simulink model "DWT_opt_fixed_point"  (R2022b)
settings: Solver=VariableStepAuto  StartTime=0.0  StopTime=st*279+st*length(signalx)  RelTol=1e-3
undefined symbols (not defined in the file): st, xc7z020clg484
libraries: hdlBasic x690, vmcUtilities x1
(part 1 of 3)
settings Model: Creator=SHMLab  LastModifiedBy=alanh

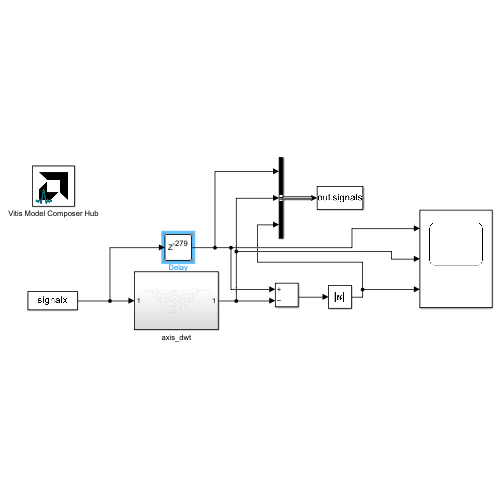
[thumbnail: Simulink's stored preview of the top-level diagram]
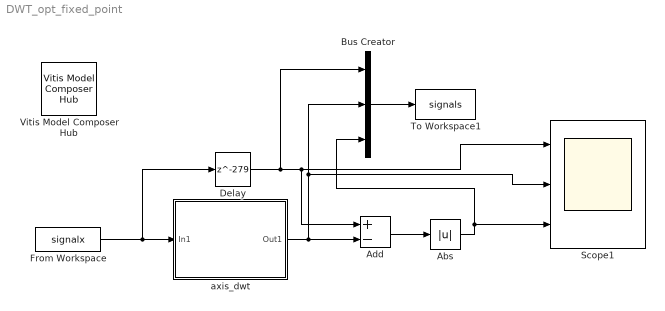
== system DWT_opt_fixed_point ==
  Abs : Abs  SaturateOnIntegerOverflow=off
  Add : Sum  Inputs=+-
  Bus Creator : BusCreator  Inputs=3
  Delay : Delay  DelayLength=279  InitialCondition=0
  From Workspace : FromWorkspace  VariableName=signalx  SampleTime=st  Interpolate=off  OutputAfterFinalValue=Setting to zero
  Scope1 : Scope  NumInputPorts=3
  To Workspace1 : ToWorkspace  VariableName=signals  SaveFormat=Timeseries  SampleTime=-1
      settings: Save2DSignal=2-D array (concatenate along first dimension)
  Vitis Model Composer Hub : vmcUtilities/Vitis Model Composer Hub  Tag=genX  CodeGeneration=off  SubsystemName=axis_dwt  TargetDirectory=./code  ExportType=HDL  IpVendor=xilinx.com  IpLibrary=hls  IpVersion=1.0  IpHWLanguage=Verilog  AieCompilerOptions={}  AieSimulatorOptions={}  CreateTestbench=off  TestbenchStackSize=10  RunRtlSim=off  RunCSim=off  RunAieSim=off  AieSimTimeout=50000  RunAieSimProfiling=off  LaunchVitisAnalyzer=off  PlotOutput=off  RunX86Sim=off  X86SimTimeout=10  GenHwImage=off  GenLibadfXo=off  PlatformType=Not Specified  HwSystemType=Baremetal  HwValidationTarget=hw  ProjDevice=xc7z020clg484-1  ProjDevicePart=xc7z020clg484-1  AIEType=None  SamplePeriod=-1  ClockFrequency=200  DataPathParallelism=1  xilinxfamily=zynq  part=xc7z020  speed=-1  package=clg484  directory=C:/Users/alanh/Downloads/Thesis/vivado/ip_with_clk_en\ip\axis_dwt\src  testbench=off  incr_netlist=off  synthesis_tool=Vivado  clock_wrapper=Clock Enables  dbl_ovrd=According to Block Masks  dcm_input_clock_period=10  sysclk_period=10  simulink_period=st  eval_field=0  IPInfoJsonString="{\"HDLSubsystem\":{\"SubsystemName\":\"axis_dwt\",\"IPName\":\"DWT\",\"IPLibrary\":\"VMC\",\"IPVendor\":\"User Company\",\"IPVersion\":\"1.0\",\"TargetDirectory\":\"C:/Users/alanh/Downloads/Thesis/vivado/ip_with_clk_en\",\"SubsystemDir\":\"C:/Users/alanh/Downloads/Thesis/vivado/ip_with_clk_en\\\\ip\\\\axis_dwt\"}}"  LogFileName=''  NThreads=4
  axis_dwt : Subsystem
  wires:
  axis_dwt/1(Out1) -> Bus Creator/2, Scope1/2, Add/2
  Delay/1 -> Scope1/1, Add/1, Bus Creator/1
  Add/1 -> Abs/1
  From Workspace/1 -> axis_dwt/1(In1), Delay/1
  Abs/1 -> Bus Creator/3, Scope1/3
  Bus Creator/1 -> To Workspace1/1

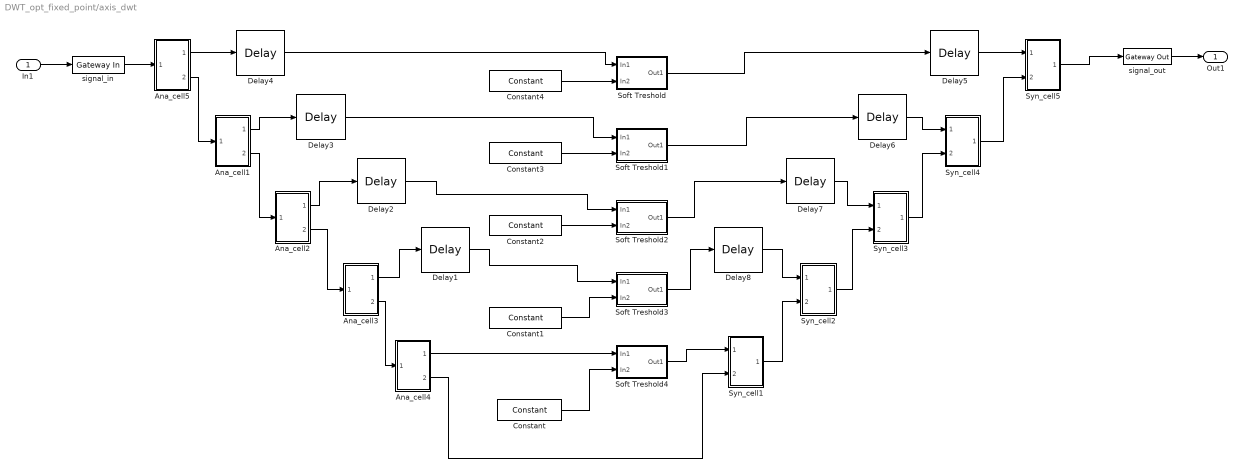
== system DWT_opt_fixed_point/axis_dwt ==
  In1 : Inport
  Ana_cell1 : Subsystem
  Ana_cell2 : Subsystem
  Ana_cell3 : Subsystem
  Ana_cell4 : Subsystem
  Ana_cell5 : Subsystem
  Constant : hdlBasic/Constant  const=0.0737  gui_display_data_type=Fixed-point  arith_type=Signed (2's comp)  n_bits=16  bin_pt=14  preci_type=Single  exp_width=8  frac_width=24  explicit_period=off  period=1  XmcBlockStatus=1  maskContainerNames=tabcontainer1  block_type=constant  block_config=sysgen:Constant_config
  Constant1 : hdlBasic/Constant  const=0.0257  gui_display_data_type=Fixed-point  arith_type=Signed (2's comp)  n_bits=16  bin_pt=14  preci_type=Single  exp_width=8  frac_width=24  explicit_period=off  period=1  XmcBlockStatus=1  maskContainerNames=tabcontainer1  block_type=constant  block_config=sysgen:Constant_config
  Constant2 : hdlBasic/Constant  const=0.0263  gui_display_data_type=Fixed-point  arith_type=Signed (2's comp)  n_bits=16  bin_pt=14  preci_type=Single  exp_width=8  frac_width=24  explicit_period=off  period=1  XmcBlockStatus=1  maskContainerNames=tabcontainer1  block_type=constant  block_config=sysgen:Constant_config
  Constant3 : hdlBasic/Constant  const=0.0053  gui_display_data_type=Fixed-point  arith_type=Signed (2's comp)  n_bits=16  bin_pt=14  preci_type=Single  exp_width=8  frac_width=24  explicit_period=off  period=1  XmcBlockStatus=1  maskContainerNames=tabcontainer1  block_type=constant  block_config=sysgen:Constant_config
  Constant4 : hdlBasic/Constant  const=0.0015  gui_display_data_type=Fixed-point  arith_type=Signed (2's comp)  n_bits=16  bin_pt=14  preci_type=Single  exp_width=8  frac_width=24  explicit_period=off  period=1  XmcBlockStatus=1  maskContainerNames=tabcontainer1  block_type=constant  block_config=sysgen:Constant_config
  Delay1 : hdlBasic/Delay  rst=off  en=off  latency=4  reg_retiming=off  XmcBlockStatus=1  maskContainerNames=group1  block_type=delay  block_config=sysgen:Delay_config
  Delay2 : hdlBasic/Delay  rst=off  en=off  latency=13  reg_retiming=off  XmcBlockStatus=1  maskContainerNames=group1  block_type=delay  block_config=sysgen:Delay_config
  Delay3 : hdlBasic/Delay  rst=off  en=off  latency=31  reg_retiming=off  XmcBlockStatus=1  maskContainerNames=group1  block_type=delay  block_config=sysgen:Delay_config
  Delay4 : hdlBasic/Delay  rst=off  en=off  latency=67  reg_retiming=off  XmcBlockStatus=1  maskContainerNames=group1  block_type=delay  block_config=sysgen:Delay_config
  Delay5 : hdlBasic/Delay  rst=off  en=off  latency=68  reg_retiming=off  XmcBlockStatus=1  maskContainerNames=group1  block_type=delay  block_config=sysgen:Delay_config
  Delay6 : hdlBasic/Delay  rst=off  en=off  latency=32  reg_retiming=off  XmcBlockStatus=1  maskContainerNames=group1  block_type=delay  block_config=sysgen:Delay_config
  Delay7 : hdlBasic/Delay  rst=off  en=off  latency=14  reg_retiming=off  XmcBlockStatus=1  maskContainerNames=group1  block_type=delay  block_config=sysgen:Delay_config
  Delay8 : hdlBasic/Delay  rst=off  en=off  latency=5  reg_retiming=off  XmcBlockStatus=1  maskContainerNames=group1  block_type=delay  block_config=sysgen:Delay_config
  Soft Treshold : Subsystem
  Soft Treshold1 : Subsystem
  Soft Treshold2 : Subsystem
  Soft Treshold3 : Subsystem
  Soft Treshold4 : Subsystem
  Syn_cell1 : Subsystem
  Syn_cell2 : Subsystem
  Syn_cell3 : Subsystem
  Syn_cell4 : Subsystem
  Syn_cell5 : Subsystem
  signal_in : hdlBasic/Gateway In  gui_display_data_type=Fixed-point  arith_type=Signed (2's comp)  n_bits=18  bin_pt=16  preci_type=Single  exp_width=8  frac_width=24  rows=1  columns=1  quantization=Truncate  overflow=Wrap  period=st  UseAsADC=off  ADCChannel='1'  interface=None  automatic_assignment=on  address_offset=hex2dec('00')  intf_name='input_signal'  intf_description=''  default_value=0  timing_constraint=Data Rate  locs_specified=off  LOCs={}  io_standard={}  inherit_from_input=off  hdl_port=on  XmcBlockStatus=1  maskContainerNames=group4  block_type=gatewayin  block_config=sysgen:gateway_in_config  block_width_w=590  block_height_w=620  block_width=640  block_height=850
  signal_out : hdlBasic/Gateway Out  inherit_from_input=off  hdl_port=on  rows=1  columns=1  UseAsDAC=off  DACChannel='1'  interface=None  automatic_assignment=on  address_offset=hex2dec('00')  intf_name='output_signal'  intf_description=''  timing_constraint=Data Rate  locs_specified=off  LOCs={}  io_standard={}  XmcBlockStatus=1  maskContainerNames=group4  block_type=gatewayout  block_config=sysgen:gateway_out_config  block_width_w=590  block_height_w=620  block_width=620  block_height=750
  Out1 : Outport
  wires:
  In1/1 -> signal_in/1
  Delay1/1 -> Soft Treshold3/1(In1)
  Soft Treshold1/1(Out1) -> Delay6/1
  Constant2/1 -> Soft Treshold2/2(In2)
  Ana_cell4/1(Out1) -> Soft Treshold4/1(In1)
  Soft Treshold4/1(Out1) -> Syn_cell1/1(In1)
  Delay6/1 -> Syn_cell4/1(In1)
  Ana_cell3/1(Out1) -> Delay1/1
  Ana_cell3/2(Out2) -> Ana_cell4/1(In1)
  Constant3/1 -> Soft Treshold1/2(In2)
  Ana_cell5/2(Out2) -> Ana_cell1/1(In1)
  Soft Treshold/1(Out1) -> Delay5/1
  Constant1/1 -> Soft Treshold3/2(In2)
  Constant/1 -> Soft Treshold4/2(In2)
  Ana_cell5/1(Out1) -> Delay4/1
  Syn_cell2/1(Out1) -> Syn_cell3/2(In2)
  Delay8/1 -> Syn_cell2/1(In1)
  Ana_cell2/1(Out1) -> Delay2/1
  signal_in/1 -> Ana_cell5/1(In1)
  Ana_cell2/2(Out2) -> Ana_cell3/1(In1)
  Ana_cell4/2(Out2) -> Syn_cell1/2(In2)
  Ana_cell1/2(Out2) -> Ana_cell2/1(In1)
  Syn_cell4/1(Out1) -> Syn_cell5/2(In2)
  Delay7/1 -> Syn_cell3/1(In1)
  Syn_cell1/1(Out1) -> Syn_cell2/2(In2)
  signal_out/1 -> Out1/1
  Soft Treshold3/1(Out1) -> Delay8/1
  Delay5/1 -> Syn_cell5/1(In1)
  Ana_cell1/1(Out1) -> Delay3/1
  Syn_cell5/1(Out1) -> signal_out/1
  Syn_cell3/1(Out1) -> Syn_cell4/2(In2)
  Delay2/1 -> Soft Treshold2/1(In1)
  Delay3/1 -> Soft Treshold1/1(In1)
  Soft Treshold2/1(Out1) -> Delay7/1
  Delay4/1 -> Soft Treshold/1(In1)
  Constant4/1 -> Soft Treshold/2(In2)

== system DWT_opt_fixed_point/axis_dwt/Ana_cell1 ==
  In1 : Inport
  D_HI : Subsystem
  D_LO : Subsystem
  Down Sample : hdlBasic/Down Sample  sample_ratio=2  sample_phase="Last Value of Frame  (most efficient)"  en=off  rst=off  latency=1  XmcBlockStatus=1  maskContainerNames=group1  block_type=dsamp  block_config=sysgen:Downsample_config
  Down Sample1 : hdlBasic/Down Sample  sample_ratio=2  sample_phase="Last Value of Frame  (most efficient)"  en=off  rst=off  latency=1  XmcBlockStatus=1  maskContainerNames=group1  block_type=dsamp  block_config=sysgen:Downsample_config
  Out1 : Outport
  Out2 : Outport  Port=2
  wires:
  D_HI/1(Out1) -> Down Sample1/1
  In1/1 -> D_LO/1(In1), D_HI/1(In1)
  D_LO/1(Out1) -> Down Sample/1
  Down Sample1/1 -> Out1/1
  Down Sample/1 -> Out2/1

== system DWT_opt_fixed_point/axis_dwt/Ana_cell2 ==
  In1 : Inport
  D_HI : Subsystem
  D_LO : Subsystem
  Down Sample : hdlBasic/Down Sample  sample_ratio=2  sample_phase="Last Value of Frame  (most efficient)"  en=off  rst=off  latency=1  XmcBlockStatus=1  maskContainerNames=group1  block_type=dsamp  block_config=sysgen:Downsample_config
  Down Sample1 : hdlBasic/Down Sample  sample_ratio=2  sample_phase="Last Value of Frame  (most efficient)"  en=off  rst=off  latency=1  XmcBlockStatus=1  maskContainerNames=group1  block_type=dsamp  block_config=sysgen:Downsample_config
  Out1 : Outport
  Out2 : Outport  Port=2
  wires:
  D_HI/1(Out1) -> Down Sample1/1
  In1/1 -> D_LO/1(In1), D_HI/1(In1)
  D_LO/1(Out1) -> Down Sample/1
  Down Sample1/1 -> Out1/1
  Down Sample/1 -> Out2/1

== system DWT_opt_fixed_point/axis_dwt/Ana_cell3 ==
  In1 : Inport
  D_HI : Subsystem
  D_LO : Subsystem
  Down Sample : hdlBasic/Down Sample  sample_ratio=2  sample_phase="Last Value of Frame  (most efficient)"  en=off  rst=off  latency=1  XmcBlockStatus=1  maskContainerNames=group1  block_type=dsamp  block_config=sysgen:Downsample_config
  Down Sample1 : hdlBasic/Down Sample  sample_ratio=2  sample_phase="Last Value of Frame  (most efficient)"  en=off  rst=off  latency=1  XmcBlockStatus=1  maskContainerNames=group1  block_type=dsamp  block_config=sysgen:Downsample_config
  Out1 : Outport
  Out2 : Outport  Port=2
  wires:
  D_HI/1(Out1) -> Down Sample1/1
  In1/1 -> D_LO/1(In1), D_HI/1(In1)
  D_LO/1(Out1) -> Down Sample/1
  Down Sample1/1 -> Out1/1
  Down Sample/1 -> Out2/1

== system DWT_opt_fixed_point/axis_dwt/Ana_cell4 ==
  In1 : Inport
  D_HI : Subsystem
  D_LO : Subsystem
  Down Sample : hdlBasic/Down Sample  sample_ratio=2  sample_phase="Last Value of Frame  (most efficient)"  en=off  rst=off  latency=1  XmcBlockStatus=1  maskContainerNames=group1  block_type=dsamp  block_config=sysgen:Downsample_config
  Down Sample1 : hdlBasic/Down Sample  sample_ratio=2  sample_phase="Last Value of Frame  (most efficient)"  en=off  rst=off  latency=1  XmcBlockStatus=1  maskContainerNames=group1  block_type=dsamp  block_config=sysgen:Downsample_config
  Out1 : Outport
  Out2 : Outport  Port=2
  wires:
  D_HI/1(Out1) -> Down Sample1/1
  In1/1 -> D_LO/1(In1), D_HI/1(In1)
  D_LO/1(Out1) -> Down Sample/1
  Down Sample1/1 -> Out1/1
  Down Sample/1 -> Out2/1

== system DWT_opt_fixed_point/axis_dwt/Ana_cell5 ==
  In1 : Inport
  D_HI : Subsystem
  D_LO : Subsystem
  Down Sample : hdlBasic/Down Sample  sample_ratio=2  sample_phase="Last Value of Frame  (most efficient)"  en=off  rst=off  latency=1  XmcBlockStatus=1  maskContainerNames=group1  block_type=dsamp  block_config=sysgen:Downsample_config
  Down Sample1 : hdlBasic/Down Sample  sample_ratio=2  sample_phase="Last Value of Frame  (most efficient)"  en=off  rst=off  latency=1  XmcBlockStatus=1  maskContainerNames=group1  block_type=dsamp  block_config=sysgen:Downsample_config
  Out1 : Outport
  Out2 : Outport  Port=2
  wires:
  D_HI/1(Out1) -> Down Sample1/1
  In1/1 -> D_LO/1(In1), D_HI/1(In1)
  D_LO/1(Out1) -> Down Sample/1
  Down Sample1/1 -> Out1/1
  Down Sample/1 -> Out2/1

== system DWT_opt_fixed_point/axis_dwt/Soft Treshold ==
  In1 : Inport
  In2 : Inport  Port=2
  AddSub : hdlBasic/AddSub  mode=Addition  use_carryin=off  use_carryout=off  en=off  latency=0  precision=User Defined  arith_type="Signed  (2's comp)"  n_bits=18  bin_pt=16  quantization=Truncate  overflow=Wrap  use_behavioral_HDL=off  hw_selection=Fabric  pipelined=off  XmcBlockStatus=1  maskContainerNames=tabcontainer1  block_type=addsub  block_config=sysgen:Addsub_config
  AddSub1 : hdlBasic/AddSub  mode=Subtraction  use_carryin=off  use_carryout=off  en=off  latency=0  precision=User Defined  arith_type="Signed  (2's comp)"  n_bits=18  bin_pt=16  quantization=Truncate  overflow=Wrap  use_behavioral_HDL=off  hw_selection=Fabric  pipelined=off  XmcBlockStatus=1  maskContainerNames=tabcontainer1  block_type=addsub  block_config=sysgen:Addsub_config
  AddSub2 : hdlBasic/AddSub  mode=Addition  use_carryin=off  use_carryout=off  en=off  latency=0  precision=User Defined  arith_type="Signed  (2's comp)"  n_bits=18  bin_pt=16  quantization=Truncate  overflow=Wrap  use_behavioral_HDL=off  hw_selection=Fabric  pipelined=off  XmcBlockStatus=1  maskContainerNames=tabcontainer1  block_type=addsub  block_config=sysgen:Addsub_config
  Constant : hdlBasic/Constant  const=0  gui_display_data_type=Fixed-point  arith_type=Signed (2's comp)  n_bits=16  bin_pt=14  preci_type=Single  exp_width=8  frac_width=24  explicit_period=off  period=1  XmcBlockStatus=1  maskContainerNames=tabcontainer1  block_type=constant  block_config=sysgen:Constant_config
  Mux : hdlBasic/Mux  inputs=2  en=off  latency=0  precision=Full  arith_type=Unsigned  n_bits=16  bin_pt=14  quantization=Truncate  overflow=Wrap  XmcBlockStatus=1  maskContainerNames=tabcontainer1  block_type=mux  block_config=sysgen:Mux_config
  Mux1 : hdlBasic/Mux  inputs=2  en=off  latency=0  precision=Full  arith_type=Unsigned  n_bits=16  bin_pt=14  quantization=Truncate  overflow=Wrap  XmcBlockStatus=1  maskContainerNames=tabcontainer1  block_type=mux  block_config=sysgen:Mux_config
  Negate : hdlBasic/Negate  precision=Full  arith_type=Unsigned  n_bits=16  bin_pt=14  quantization=Truncate  overflow=Wrap  en=off  latency=0  XmcBlockStatus=1  maskContainerNames=tabcontainer1  block_type=negate  block_config=sysgen:Negate_config
  Relational : hdlBasic/Relational  mode=a>b  op_type=Bool  en=off  latency=0  XmcBlockStatus=1  maskContainerNames=tabcontainer1  block_type=relational  block_config=sysgen:Relational_config
  Relational1 : hdlBasic/Relational  mode=a<b  op_type=Bool  en=off  latency=0  XmcBlockStatus=1  maskContainerNames=tabcontainer1  block_type=relational  block_config=sysgen:Relational_config
  Out1 : Outport
  wires:
  AddSub/1 -> Mux1/3
  Constant/1 -> Mux1/2, Mux/2
  Relational/1 -> Mux/1
  Mux1/1 -> AddSub2/2
  In1/1 -> AddSub/1, Relational1/1, AddSub1/1, Relational/1
  Mux/1 -> AddSub2/1
  In2/1 -> AddSub/2, Negate/1, AddSub1/2, Relational/2
  AddSub1/1 -> Mux/3
  Relational1/1 -> Mux1/1
  Negate/1 -> Relational1/2
  AddSub2/1 -> Out1/1

== system DWT_opt_fixed_point/axis_dwt/Soft Treshold1 ==
  In1 : Inport
  In2 : Inport  Port=2
  AddSub : hdlBasic/AddSub  mode=Addition  use_carryin=off  use_carryout=off  en=off  latency=0  precision=User Defined  arith_type="Signed  (2's comp)"  n_bits=18  bin_pt=16  quantization=Truncate  overflow=Wrap  use_behavioral_HDL=off  hw_selection=Fabric  pipelined=off  XmcBlockStatus=1  maskContainerNames=tabcontainer1  block_type=addsub  block_config=sysgen:Addsub_config
  AddSub1 : hdlBasic/AddSub  mode=Subtraction  use_carryin=off  use_carryout=off  en=off  latency=0  precision=User Defined  arith_type="Signed  (2's comp)"  n_bits=18  bin_pt=16  quantization=Truncate  overflow=Wrap  use_behavioral_HDL=off  hw_selection=Fabric  pipelined=off  XmcBlockStatus=1  maskContainerNames=tabcontainer1  block_type=addsub  block_config=sysgen:Addsub_config
  AddSub2 : hdlBasic/AddSub  mode=Addition  use_carryin=off  use_carryout=off  en=off  latency=0  precision=User Defined  arith_type="Signed  (2's comp)"  n_bits=18  bin_pt=16  quantization=Truncate  overflow=Wrap  use_behavioral_HDL=off  hw_selection=Fabric  pipelined=off  XmcBlockStatus=1  maskContainerNames=tabcontainer1  block_type=addsub  block_config=sysgen:Addsub_config
  Constant : hdlBasic/Constant  const=0  gui_display_data_type=Fixed-point  arith_type=Signed (2's comp)  n_bits=16  bin_pt=14  preci_type=Single  exp_width=8  frac_width=24  explicit_period=off  period=1  XmcBlockStatus=1  maskContainerNames=tabcontainer1  block_type=constant  block_config=sysgen:Constant_config
  Mux : hdlBasic/Mux  inputs=2  en=off  latency=0  precision=Full  arith_type=Unsigned  n_bits=16  bin_pt=14  quantization=Truncate  overflow=Wrap  XmcBlockStatus=1  maskContainerNames=tabcontainer1  block_type=mux  block_config=sysgen:Mux_config
  Mux1 : hdlBasic/Mux  inputs=2  en=off  latency=0  precision=Full  arith_type=Unsigned  n_bits=16  bin_pt=14  quantization=Truncate  overflow=Wrap  XmcBlockStatus=1  maskContainerNames=tabcontainer1  block_type=mux  block_config=sysgen:Mux_config
  Negate : hdlBasic/Negate  precision=Full  arith_type=Unsigned  n_bits=16  bin_pt=14  quantization=Truncate  overflow=Wrap  en=off  latency=0  XmcBlockStatus=1  maskContainerNames=tabcontainer1  block_type=negate  block_config=sysgen:Negate_config
  Relational : hdlBasic/Relational  mode=a>b  op_type=Bool  en=off  latency=0  XmcBlockStatus=1  maskContainerNames=tabcontainer1  block_type=relational  block_config=sysgen:Relational_config
  Relational1 : hdlBasic/Relational  mode=a<b  op_type=Bool  en=off  latency=0  XmcBlockStatus=1  maskContainerNames=tabcontainer1  block_type=relational  block_config=sysgen:Relational_config
  Out1 : Outport
  wires:
  AddSub/1 -> Mux1/3
  Constant/1 -> Mux1/2, Mux/2
  Relational/1 -> Mux/1
  Mux1/1 -> AddSub2/2
  In1/1 -> AddSub/1, Relational1/1, AddSub1/1, Relational/1
  Mux/1 -> AddSub2/1
  In2/1 -> AddSub/2, Negate/1, AddSub1/2, Relational/2
  AddSub1/1 -> Mux/3
  Relational1/1 -> Mux1/1
  Negate/1 -> Relational1/2
  AddSub2/1 -> Out1/1

== system DWT_opt_fixed_point/axis_dwt/Soft Treshold2 ==
  In1 : Inport
  In2 : Inport  Port=2
  AddSub : hdlBasic/AddSub  mode=Addition  use_carryin=off  use_carryout=off  en=off  latency=0  precision=User Defined  arith_type="Signed  (2's comp)"  n_bits=18  bin_pt=16  quantization=Truncate  overflow=Wrap  use_behavioral_HDL=off  hw_selection=Fabric  pipelined=off  XmcBlockStatus=1  maskContainerNames=tabcontainer1  block_type=addsub  block_config=sysgen:Addsub_config
  AddSub1 : hdlBasic/AddSub  mode=Subtraction  use_carryin=off  use_carryout=off  en=off  latency=0  precision=User Defined  arith_type="Signed  (2's comp)"  n_bits=18  bin_pt=16  quantization=Truncate  overflow=Wrap  use_behavioral_HDL=off  hw_selection=Fabric  pipelined=off  XmcBlockStatus=1  maskContainerNames=tabcontainer1  block_type=addsub  block_config=sysgen:Addsub_config
  AddSub2 : hdlBasic/AddSub  mode=Addition  use_carryin=off  use_carryout=off  en=off  latency=0  precision=User Defined  arith_type="Signed  (2's comp)"  n_bits=18  bin_pt=16  quantization=Truncate  overflow=Wrap  use_behavioral_HDL=off  hw_selection=Fabric  pipelined=off  XmcBlockStatus=1  maskContainerNames=tabcontainer1  block_type=addsub  block_config=sysgen:Addsub_config
  Constant : hdlBasic/Constant  const=0  gui_display_data_type=Fixed-point  arith_type=Signed (2's comp)  n_bits=16  bin_pt=14  preci_type=Single  exp_width=8  frac_width=24  explicit_period=off  period=1  XmcBlockStatus=1  maskContainerNames=tabcontainer1  block_type=constant  block_config=sysgen:Constant_config
  Mux : hdlBasic/Mux  inputs=2  en=off  latency=0  precision=Full  arith_type=Unsigned  n_bits=16  bin_pt=14  quantization=Truncate  overflow=Wrap  XmcBlockStatus=1  maskContainerNames=tabcontainer1  block_type=mux  block_config=sysgen:Mux_config
  Mux1 : hdlBasic/Mux  inputs=2  en=off  latency=0  precision=Full  arith_type=Unsigned  n_bits=16  bin_pt=14  quantization=Truncate  overflow=Wrap  XmcBlockStatus=1  maskContainerNames=tabcontainer1  block_type=mux  block_config=sysgen:Mux_config
  Negate : hdlBasic/Negate  precision=Full  arith_type=Unsigned  n_bits=16  bin_pt=14  quantization=Truncate  overflow=Wrap  en=off  latency=0  XmcBlockStatus=1  maskContainerNames=tabcontainer1  block_type=negate  block_config=sysgen:Negate_config
  Relational : hdlBasic/Relational  mode=a>b  op_type=Bool  en=off  latency=0  XmcBlockStatus=1  maskContainerNames=tabcontainer1  block_type=relational  block_config=sysgen:Relational_config
  Relational1 : hdlBasic/Relational  mode=a<b  op_type=Bool  en=off  latency=0  XmcBlockStatus=1  maskContainerNames=tabcontainer1  block_type=relational  block_config=sysgen:Relational_config
  Out1 : Outport
  wires:
  AddSub/1 -> Mux1/3
  Constant/1 -> Mux1/2, Mux/2
  Relational/1 -> Mux/1
  Mux1/1 -> AddSub2/2
  In1/1 -> AddSub/1, Relational1/1, AddSub1/1, Relational/1
  Mux/1 -> AddSub2/1
  In2/1 -> AddSub/2, Negate/1, AddSub1/2, Relational/2
  AddSub1/1 -> Mux/3
  Relational1/1 -> Mux1/1
  Negate/1 -> Relational1/2
  AddSub2/1 -> Out1/1

== system DWT_opt_fixed_point/axis_dwt/Soft Treshold3 ==
  In1 : Inport
  In2 : Inport  Port=2
  AddSub : hdlBasic/AddSub  mode=Addition  use_carryin=off  use_carryout=off  en=off  latency=0  precision=User Defined  arith_type="Signed  (2's comp)"  n_bits=18  bin_pt=16  quantization=Truncate  overflow=Wrap  use_behavioral_HDL=off  hw_selection=Fabric  pipelined=off  XmcBlockStatus=1  maskContainerNames=tabcontainer1  block_type=addsub  block_config=sysgen:Addsub_config
  AddSub1 : hdlBasic/AddSub  mode=Subtraction  use_carryin=off  use_carryout=off  en=off  latency=0  precision=User Defined  arith_type="Signed  (2's comp)"  n_bits=18  bin_pt=16  quantization=Truncate  overflow=Wrap  use_behavioral_HDL=off  hw_selection=Fabric  pipelined=off  XmcBlockStatus=1  maskContainerNames=tabcontainer1  block_type=addsub  block_config=sysgen:Addsub_config
  AddSub2 : hdlBasic/AddSub  mode=Addition  use_carryin=off  use_carryout=off  en=off  latency=0  precision=User Defined  arith_type="Signed  (2's comp)"  n_bits=18  bin_pt=16  quantization=Truncate  overflow=Wrap  use_behavioral_HDL=off  hw_selection=Fabric  pipelined=off  XmcBlockStatus=1  maskContainerNames=tabcontainer1  block_type=addsub  block_config=sysgen:Addsub_config
  Constant : hdlBasic/Constant  const=0  gui_display_data_type=Fixed-point  arith_type=Signed (2's comp)  n_bits=16  bin_pt=14  preci_type=Single  exp_width=8  frac_width=24  explicit_period=off  period=1  XmcBlockStatus=1  maskContainerNames=tabcontainer1  block_type=constant  block_config=sysgen:Constant_config
  Mux : hdlBasic/Mux  inputs=2  en=off  latency=0  precision=Full  arith_type=Unsigned  n_bits=16  bin_pt=14  quantization=Truncate  overflow=Wrap  XmcBlockStatus=1  maskContainerNames=tabcontainer1  block_type=mux  block_config=sysgen:Mux_config
  Mux1 : hdlBasic/Mux  inputs=2  en=off  latency=0  precision=Full  arith_type=Unsigned  n_bits=16  bin_pt=14  quantization=Truncate  overflow=Wrap  XmcBlockStatus=1  maskContainerNames=tabcontainer1  block_type=mux  block_config=sysgen:Mux_config
  Negate : hdlBasic/Negate  precision=Full  arith_type=Unsigned  n_bits=16  bin_pt=14  quantization=Truncate  overflow=Wrap  en=off  latency=0  XmcBlockStatus=1  maskContainerNames=tabcontainer1  block_type=negate  block_config=sysgen:Negate_config
  Relational : hdlBasic/Relational  mode=a>b  op_type=Bool  en=off  latency=0  XmcBlockStatus=1  maskContainerNames=tabcontainer1  block_type=relational  block_config=sysgen:Relational_config
  Relational1 : hdlBasic/Relational  mode=a<b  op_type=Bool  en=off  latency=0  XmcBlockStatus=1  maskContainerNames=tabcontainer1  block_type=relational  block_config=sysgen:Relational_config
  Out1 : Outport
  wires:
  AddSub/1 -> Mux1/3
  Constant/1 -> Mux1/2, Mux/2
  Relational/1 -> Mux/1
  Mux1/1 -> AddSub2/2
  In1/1 -> AddSub/1, Relational1/1, AddSub1/1, Relational/1
  Mux/1 -> AddSub2/1
  In2/1 -> AddSub/2, Negate/1, AddSub1/2, Relational/2
  AddSub1/1 -> Mux/3
  Relational1/1 -> Mux1/1
  Negate/1 -> Relational1/2
  AddSub2/1 -> Out1/1

== system DWT_opt_fixed_point/axis_dwt/Soft Treshold4 ==
  In1 : Inport
  In2 : Inport  Port=2
  AddSub : hdlBasic/AddSub  mode=Addition  use_carryin=off  use_carryout=off  en=off  latency=0  precision=User Defined  arith_type="Signed  (2's comp)"  n_bits=18  bin_pt=16  quantization=Truncate  overflow=Wrap  use_behavioral_HDL=off  hw_selection=Fabric  pipelined=off  XmcBlockStatus=1  maskContainerNames=tabcontainer1  block_type=addsub  block_config=sysgen:Addsub_config
  AddSub1 : hdlBasic/AddSub  mode=Subtraction  use_carryin=off  use_carryout=off  en=off  latency=0  precision=User Defined  arith_type="Signed  (2's comp)"  n_bits=18  bin_pt=16  quantization=Truncate  overflow=Wrap  use_behavioral_HDL=off  hw_selection=Fabric  pipelined=off  XmcBlockStatus=1  maskContainerNames=tabcontainer1  block_type=addsub  block_config=sysgen:Addsub_config
  AddSub2 : hdlBasic/AddSub  mode=Addition  use_carryin=off  use_carryout=off  en=off  latency=0  precision=User Defined  arith_type="Signed  (2's comp)"  n_bits=18  bin_pt=16  quantization=Truncate  overflow=Wrap  use_behavioral_HDL=off  hw_selection=Fabric  pipelined=off  XmcBlockStatus=1  maskContainerNames=tabcontainer1  block_type=addsub  block_config=sysgen:Addsub_config
  Constant : hdlBasic/Constant  const=0  gui_display_data_type=Fixed-point  arith_type=Signed (2's comp)  n_bits=16  bin_pt=14  preci_type=Single  exp_width=8  frac_width=24  explicit_period=off  period=1  XmcBlockStatus=1  maskContainerNames=tabcontainer1  block_type=constant  block_config=sysgen:Constant_config
  Mux : hdlBasic/Mux  inputs=2  en=off  latency=0  precision=Full  arith_type=Unsigned  n_bits=16  bin_pt=14  quantization=Truncate  overflow=Wrap  XmcBlockStatus=1  maskContainerNames=tabcontainer1  block_type=mux  block_config=sysgen:Mux_config
  Mux1 : hdlBasic/Mux  inputs=2  en=off  latency=0  precision=Full  arith_type=Unsigned  n_bits=16  bin_pt=14  quantization=Truncate  overflow=Wrap  XmcBlockStatus=1  maskContainerNames=tabcontainer1  block_type=mux  block_config=sysgen:Mux_config
  Negate : hdlBasic/Negate  precision=Full  arith_type=Unsigned  n_bits=16  bin_pt=14  quantization=Truncate  overflow=Wrap  en=off  latency=0  XmcBlockStatus=1  maskContainerNames=tabcontainer1  block_type=negate  block_config=sysgen:Negate_config
  Relational : hdlBasic/Relational  mode=a>b  op_type=Bool  en=off  latency=0  XmcBlockStatus=1  maskContainerNames=tabcontainer1  block_type=relational  block_config=sysgen:Relational_config
  Relational1 : hdlBasic/Relational  mode=a<b  op_type=Bool  en=off  latency=0  XmcBlockStatus=1  maskContainerNames=tabcontainer1  block_type=relational  block_config=sysgen:Relational_config
  Out1 : Outport
  wires:
  AddSub/1 -> Mux1/3
  Constant/1 -> Mux1/2, Mux/2
  Relational/1 -> Mux/1
  Mux1/1 -> AddSub2/2
  In1/1 -> AddSub/1, Relational1/1, AddSub1/1, Relational/1
  Mux/1 -> AddSub2/1
  In2/1 -> AddSub/2, Negate/1, AddSub1/2, Relational/2
  AddSub1/1 -> Mux/3
  Relational1/1 -> Mux1/1
  Negate/1 -> Relational1/2
  AddSub2/1 -> Out1/1

== system DWT_opt_fixed_point/axis_dwt/Syn_cell1 ==
  In1 : Inport
  In2 : Inport  Port=2
  AddSub : hdlBasic/AddSub  mode=Addition  use_carryin=off  use_carryout=off  en=off  latency=0  precision=User Defined  arith_type="Signed  (2's comp)"  n_bits=18  bin_pt=16  quantization=Truncate  overflow=Wrap  use_behavioral_HDL=off  hw_selection=Fabric  pipelined=off  XmcBlockStatus=1  maskContainerNames=tabcontainer1  block_type=addsub  block_config=sysgen:Addsub_config
  Delay : hdlBasic/Delay  rst=off  en=off  latency=1  reg_retiming=off  XmcBlockStatus=1  maskContainerNames=group1  block_type=delay  block_config=sysgen:Delay_config
  R_HI : Subsystem
  R_LO : Subsystem
  Up Sample : hdlBasic/Up Sample  sample_ratio=2  copy_samples=off  en=off  latency=0  XmcBlockStatus=1  maskContainerNames=group1  block_type=usamp  block_config=sysgen:Upsample_config
  Up Sample1 : hdlBasic/Up Sample  sample_ratio=2  copy_samples=off  en=off  latency=0  XmcBlockStatus=1  maskContainerNames=group1  block_type=usamp  block_config=sysgen:Upsample_config
  Out1 : Outport
  wires:
  R_HI/1(Out1) -> AddSub/1
  R_LO/1(Out1) -> AddSub/2
  In2/1 -> Up Sample1/1
  Up Sample1/1 -> R_LO/1(In1)
  Up Sample/1 -> R_HI/1(In1)
  In1/1 -> Up Sample/1
  AddSub/1 -> Delay/1
  Delay/1 -> Out1/1

== system DWT_opt_fixed_point/axis_dwt/Syn_cell2 ==
  In1 : Inport
  In2 : Inport  Port=2
  AddSub : hdlBasic/AddSub  mode=Addition  use_carryin=off  use_carryout=off  en=off  latency=0  precision=User Defined  arith_type="Signed  (2's comp)"  n_bits=18  bin_pt=16  quantization=Truncate  overflow=Wrap  use_behavioral_HDL=off  hw_selection=Fabric  pipelined=off  XmcBlockStatus=1  maskContainerNames=tabcontainer1  block_type=addsub  block_config=sysgen:Addsub_config
  Delay : hdlBasic/Delay  rst=off  en=off  latency=1  reg_retiming=off  XmcBlockStatus=1  maskContainerNames=group1  block_type=delay  block_config=sysgen:Delay_config
  R_HI : Subsystem
  R_LO : Subsystem
  Up Sample : hdlBasic/Up Sample  sample_ratio=2  copy_samples=off  en=off  latency=0  XmcBlockStatus=1  maskContainerNames=group1  block_type=usamp  block_config=sysgen:Upsample_config
  Up Sample1 : hdlBasic/Up Sample  sample_ratio=2  copy_samples=off  en=off  latency=0  XmcBlockStatus=1  maskContainerNames=group1  block_type=usamp  block_config=sysgen:Upsample_config
  Out1 : Outport
  wires:
  R_HI/1(Out1) -> AddSub/1
  R_LO/1(Out1) -> AddSub/2
  In2/1 -> Up Sample1/1
  Up Sample1/1 -> R_LO/1(In1)
  Up Sample/1 -> R_HI/1(In1)
  In1/1 -> Up Sample/1
  AddSub/1 -> Delay/1
  Delay/1 -> Out1/1

== system DWT_opt_fixed_point/axis_dwt/Syn_cell3 ==
  In1 : Inport
  In2 : Inport  Port=2
  AddSub : hdlBasic/AddSub  mode=Addition  use_carryin=off  use_carryout=off  en=off  latency=0  precision=User Defined  arith_type="Signed  (2's comp)"  n_bits=18  bin_pt=16  quantization=Truncate  overflow=Wrap  use_behavioral_HDL=off  hw_selection=Fabric  pipelined=off  XmcBlockStatus=1  maskContainerNames=tabcontainer1  block_type=addsub  block_config=sysgen:Addsub_config
  Delay : hdlBasic/Delay  rst=off  en=off  latency=1  reg_retiming=off  XmcBlockStatus=1  maskContainerNames=group1  block_type=delay  block_config=sysgen:Delay_config
  R_HI : Subsystem
  R_LO : Subsystem
  Up Sample : hdlBasic/Up Sample  sample_ratio=2  copy_samples=off  en=off  latency=0  XmcBlockStatus=1  maskContainerNames=group1  block_type=usamp  block_config=sysgen:Upsample_config
  Up Sample1 : hdlBasic/Up Sample  sample_ratio=2  copy_samples=off  en=off  latency=0  XmcBlockStatus=1  maskContainerNames=group1  block_type=usamp  block_config=sysgen:Upsample_config
  Out1 : Outport
  wires:
  R_HI/1(Out1) -> AddSub/1
  R_LO/1(Out1) -> AddSub/2
  In2/1 -> Up Sample1/1
  Up Sample1/1 -> R_LO/1(In1)
  Up Sample/1 -> R_HI/1(In1)
  In1/1 -> Up Sample/1
  AddSub/1 -> Delay/1
  Delay/1 -> Out1/1

== system DWT_opt_fixed_point/axis_dwt/Syn_cell4 ==
  In1 : Inport
  In2 : Inport  Port=2
  AddSub : hdlBasic/AddSub  mode=Addition  use_carryin=off  use_carryout=off  en=off  latency=0  precision=User Defined  arith_type="Signed  (2's comp)"  n_bits=18  bin_pt=16  quantization=Truncate  overflow=Wrap  use_behavioral_HDL=off  hw_selection=Fabric  pipelined=off  XmcBlockStatus=1  maskContainerNames=tabcontainer1  block_type=addsub  block_config=sysgen:Addsub_config
  Delay : hdlBasic/Delay  rst=off  en=off  latency=1  reg_retiming=off  XmcBlockStatus=1  maskContainerNames=group1  block_type=delay  block_config=sysgen:Delay_config
  R_HI : Subsystem
  R_LO : Subsystem
  Up Sample : hdlBasic/Up Sample  sample_ratio=2  copy_samples=off  en=off  latency=0  XmcBlockStatus=1  maskContainerNames=group1  block_type=usamp  block_config=sysgen:Upsample_config
  Up Sample1 : hdlBasic/Up Sample  sample_ratio=2  copy_samples=off  en=off  latency=0  XmcBlockStatus=1  maskContainerNames=group1  block_type=usamp  block_config=sysgen:Upsample_config
  Out1 : Outport
  wires:
  R_HI/1(Out1) -> AddSub/1
  R_LO/1(Out1) -> AddSub/2
  In2/1 -> Up Sample1/1
  Up Sample1/1 -> R_LO/1(In1)
  Up Sample/1 -> R_HI/1(In1)
  In1/1 -> Up Sample/1
  AddSub/1 -> Delay/1
  Delay/1 -> Out1/1

== system DWT_opt_fixed_point/axis_dwt/Syn_cell5 ==
  In1 : Inport
  In2 : Inport  Port=2
  AddSub : hdlBasic/AddSub  mode=Addition  use_carryin=off  use_carryout=off  en=off  latency=0  precision=User Defined  arith_type="Signed  (2's comp)"  n_bits=18  bin_pt=16  quantization=Truncate  overflow=Wrap  use_behavioral_HDL=off  hw_selection=Fabric  pipelined=off  XmcBlockStatus=1  maskContainerNames=tabcontainer1  block_type=addsub  block_config=sysgen:Addsub_config
  Delay : hdlBasic/Delay  rst=off  en=off  latency=1  reg_retiming=off  XmcBlockStatus=1  maskContainerNames=group1  block_type=delay  block_config=sysgen:Delay_config
  R_HI : Subsystem
  R_LO : Subsystem
  Up Sample : hdlBasic/Up Sample  sample_ratio=2  copy_samples=off  en=off  latency=0  XmcBlockStatus=1  maskContainerNames=group1  block_type=usamp  block_config=sysgen:Upsample_config
  Up Sample1 : hdlBasic/Up Sample  sample_ratio=2  copy_samples=off  en=off  latency=0  XmcBlockStatus=1  maskContainerNames=group1  block_type=usamp  block_config=sysgen:Upsample_config
  Out1 : Outport
  wires:
  R_HI/1(Out1) -> AddSub/1
  R_LO/1(Out1) -> AddSub/2
  In2/1 -> Up Sample1/1
  Up Sample1/1 -> R_LO/1(In1)
  Up Sample/1 -> R_HI/1(In1)
  In1/1 -> Up Sample/1
  AddSub/1 -> Delay/1
  Delay/1 -> Out1/1

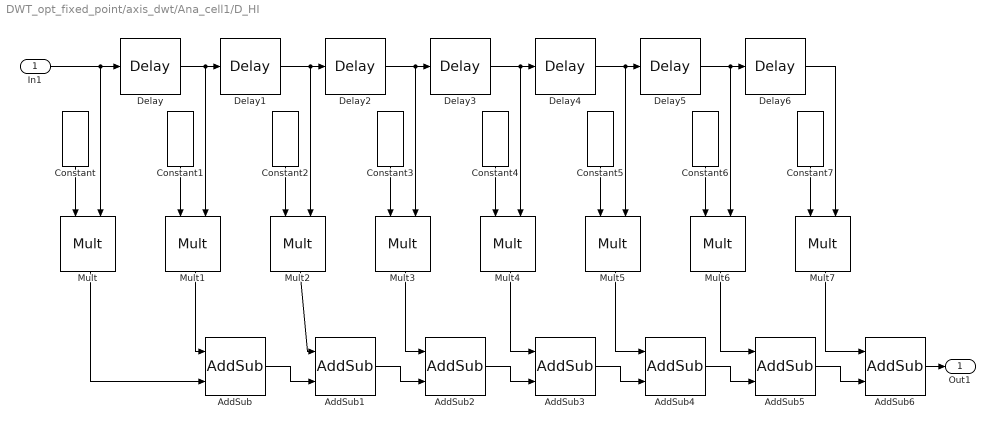
== system DWT_opt_fixed_point/axis_dwt/Ana_cell1/D_HI ==
  In1 : Inport
  AddSub{,1..6} (7 alike) : hdlBasic/AddSub  mode=Addition  use_carryin=off  use_carryout=off  en=off  latency=0  precision=User Defined  arith_type="Signed  (2's comp)"  n_bits=18  bin_pt=16  quantization=Truncate  overflow=Wrap  use_behavioral_HDL=off  hw_selection=Fabric  pipelined=off  XmcBlockStatus=1  maskContainerNames=tabcontainer1  block_type=addsub  block_config=sysgen:Addsub_config
  Constant : hdlBasic/Constant  const=-0.23037781330885523  gui_display_data_type=Fixed-point  arith_type=Signed (2's comp)  n_bits=16  bin_pt=14  preci_type=Single  exp_width=8  frac_width=24  explicit_period=off  period=1  XmcBlockStatus=1  maskContainerNames=tabcontainer1  block_type=constant  block_config=sysgen:Constant_config
  Constant1 : hdlBasic/Constant  const=0.7148465705525415  gui_display_data_type=Fixed-point  arith_type=Signed (2's comp)  n_bits=16  bin_pt=14  preci_type=Single  exp_width=8  frac_width=24  explicit_period=off  period=1  XmcBlockStatus=1  maskContainerNames=tabcontainer1  block_type=constant  block_config=sysgen:Constant_config
  Constant2 : hdlBasic/Constant  const=-0.6308807679295904  gui_display_data_type=Fixed-point  arith_type=Signed (2's comp)  n_bits=16  bin_pt=14  preci_type=Single  exp_width=8  frac_width=24  explicit_period=off  period=1  XmcBlockStatus=1  maskContainerNames=tabcontainer1  block_type=constant  block_config=sysgen:Constant_config
  Constant3 : hdlBasic/Constant  const=-0.02798376941698385  gui_display_data_type=Fixed-point  arith_type=Signed (2's comp)  n_bits=16  bin_pt=14  preci_type=Single  exp_width=8  frac_width=24  explicit_period=off  period=1  XmcBlockStatus=1  maskContainerNames=tabcontainer1  block_type=constant  block_config=sysgen:Constant_config
  Constant4 : hdlBasic/Constant  const=0.18703481171888114  gui_display_data_type=Fixed-point  arith_type=Signed (2's comp)  n_bits=16  bin_pt=14  preci_type=Single  exp_width=8  frac_width=24  explicit_period=off  period=1  XmcBlockStatus=1  maskContainerNames=tabcontainer1  block_type=constant  block_config=sysgen:Constant_config
  Constant5 : hdlBasic/Constant  const=0.030841381835986965  gui_display_data_type=Fixed-point  arith_type=Signed (2's comp)  n_bits=16  bin_pt=14  preci_type=Single  exp_width=8  frac_width=24  explicit_period=off  period=1  XmcBlockStatus=1  maskContainerNames=tabcontainer1  block_type=constant  block_config=sysgen:Constant_config
  Constant6 : hdlBasic/Constant  const=-0.032883011666982945  gui_display_data_type=Fixed-point  arith_type=Signed (2's comp)  n_bits=16  bin_pt=14  preci_type=Single  exp_width=8  frac_width=24  explicit_period=off  period=1  XmcBlockStatus=1  maskContainerNames=tabcontainer1  block_type=constant  block_config=sysgen:Constant_config
  Constant7 : hdlBasic/Constant  const=-0.010597401784997278  gui_display_data_type=Fixed-point  arith_type=Signed (2's comp)  n_bits=16  bin_pt=14  preci_type=Single  exp_width=8  frac_width=24  explicit_period=off  period=1  XmcBlockStatus=1  maskContainerNames=tabcontainer1  block_type=constant  block_config=sysgen:Constant_config
  Delay{,1..6} (7 alike) : hdlBasic/Delay  rst=off  en=off  latency=1  reg_retiming=off  XmcBlockStatus=1  maskContainerNames=group1  block_type=delay  block_config=sysgen:Delay_config
  Mult{,1..7} (8 alike) : hdlBasic/Mult  precision=User Defined  arith_type="Signed  (2's comp)"  n_bits=18  bin_pt=16  quantization=Truncate  overflow=Wrap  en=off  latency=0  use_behavioral_HDL=off  opt=Speed  use_embedded=on  optimum_pipeline=off  pipeline=on  use_rpm=on  placement_style=Triangular  XmcBlockStatus=1  maskContainerNames=group1  block_type=mult  block_config=sysgen:Mult_config  block_width=598  block_height=876
  Out1 : Outport
  wires:
  Delay3/1 -> Mult4/2, Delay4/1
  Mult2/1 -> AddSub1/1
  In1/1 -> Mult/2, Delay/1
  Constant6/1 -> Mult6/1
  Delay5/1 -> Mult6/2, Delay6/1
  Constant7/1 -> Mult7/1
  Delay1/1 -> Mult2/2, Delay2/1
  Delay/1 -> Mult1/2, Delay1/1
  AddSub6/1 -> Out1/1
  Delay2/1 -> Mult3/2, Delay3/1
  AddSub3/1 -> AddSub4/2
  Delay6/1 -> Mult7/2
  Mult3/1 -> AddSub2/1
  Constant5/1 -> Mult5/1
  AddSub/1 -> AddSub1/2
  Delay4/1 -> Mult5/2, Delay5/1
  Constant2/1 -> Mult2/1
  Mult7/1 -> AddSub6/1
  Mult1/1 -> AddSub/1
  Mult6/1 -> AddSub5/1
  AddSub4/1 -> AddSub5/2
  Mult4/1 -> AddSub3/1
  AddSub2/1 -> AddSub3/2
  Constant3/1 -> Mult3/1
  Constant/1 -> Mult/1
  Mult5/1 -> AddSub4/1
  AddSub1/1 -> AddSub2/2
  Constant4/1 -> Mult4/1
  Mult/1 -> AddSub/2
  AddSub5/1 -> AddSub6/2
  Constant1/1 -> Mult1/1

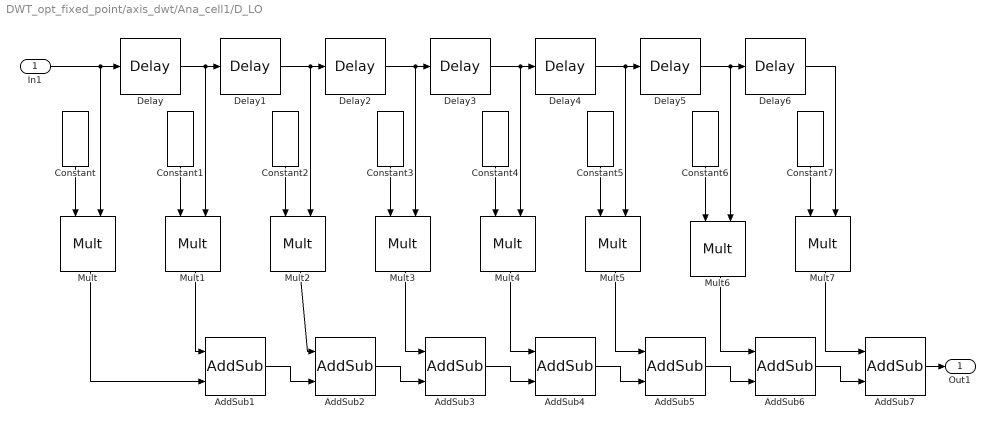
== system DWT_opt_fixed_point/axis_dwt/Ana_cell1/D_LO ==
  In1 : Inport
  AddSub{1..7} (7 alike) : hdlBasic/AddSub  mode=Addition  use_carryin=off  use_carryout=off  en=off  latency=0  precision=User Defined  arith_type="Signed  (2's comp)"  n_bits=18  bin_pt=16  quantization=Truncate  overflow=Wrap  use_behavioral_HDL=off  hw_selection=Fabric  pipelined=off  XmcBlockStatus=1  maskContainerNames=tabcontainer1  block_type=addsub  block_config=sysgen:Addsub_config
  Constant : hdlBasic/Constant  const=-0.010597401784997278  gui_display_data_type=Fixed-point  arith_type=Signed (2's comp)  n_bits=16  bin_pt=14  preci_type=Single  exp_width=8  frac_width=24  explicit_period=off  period=1  XmcBlockStatus=1  maskContainerNames=tabcontainer1  block_type=constant  block_config=sysgen:Constant_config
  Constant1 : hdlBasic/Constant  const=0.032883011666982945  gui_display_data_type=Fixed-point  arith_type=Signed (2's comp)  n_bits=16  bin_pt=14  preci_type=Single  exp_width=8  frac_width=24  explicit_period=off  period=1  XmcBlockStatus=1  maskContainerNames=tabcontainer1  block_type=constant  block_config=sysgen:Constant_config
  Constant2 : hdlBasic/Constant  const=0.030841381835986965  gui_display_data_type=Fixed-point  arith_type=Signed (2's comp)  n_bits=16  bin_pt=14  preci_type=Single  exp_width=8  frac_width=24  explicit_period=off  period=1  XmcBlockStatus=1  maskContainerNames=tabcontainer1  block_type=constant  block_config=sysgen:Constant_config
  Constant3 : hdlBasic/Constant  const=-0.18703481171888114  gui_display_data_type=Fixed-point  arith_type=Signed (2's comp)  n_bits=16  bin_pt=14  preci_type=Single  exp_width=8  frac_width=24  explicit_period=off  period=1  XmcBlockStatus=1  maskContainerNames=tabcontainer1  block_type=constant  block_config=sysgen:Constant_config
  Constant4 : hdlBasic/Constant  const=-0.02798376941698385  gui_display_data_type=Fixed-point  arith_type=Signed (2's comp)  n_bits=16  bin_pt=14  preci_type=Single  exp_width=8  frac_width=24  explicit_period=off  period=1  XmcBlockStatus=1  maskContainerNames=tabcontainer1  block_type=constant  block_config=sysgen:Constant_config
  Constant5 : hdlBasic/Constant  const=0.6308807679295904  gui_display_data_type=Fixed-point  arith_type=Signed (2's comp)  n_bits=16  bin_pt=14  preci_type=Single  exp_width=8  frac_width=24  explicit_period=off  period=1  XmcBlockStatus=1  maskContainerNames=tabcontainer1  block_type=constant  block_config=sysgen:Constant_config
  Constant6 : hdlBasic/Constant  const=0.7148465705525415  gui_display_data_type=Fixed-point  arith_type=Signed (2's comp)  n_bits=16  bin_pt=14  preci_type=Single  exp_width=8  frac_width=24  explicit_period=off  period=1  XmcBlockStatus=1  maskContainerNames=tabcontainer1  block_type=constant  block_config=sysgen:Constant_config
  Constant7 : hdlBasic/Constant  const=0.23037781330885523  gui_display_data_type=Fixed-point  arith_type=Signed (2's comp)  n_bits=16  bin_pt=14  preci_type=Single  exp_width=8  frac_width=24  explicit_period=off  period=1  XmcBlockStatus=1  maskContainerNames=tabcontainer1  block_type=constant  block_config=sysgen:Constant_config
  Delay{,1..6} (7 alike) : hdlBasic/Delay  rst=off  en=off  latency=1  reg_retiming=off  XmcBlockStatus=1  maskContainerNames=group1  block_type=delay  block_config=sysgen:Delay_config
  Mult{,1..7} (8 alike) : hdlBasic/Mult  precision=User Defined  arith_type="Signed  (2's comp)"  n_bits=18  bin_pt=16  quantization=Truncate  overflow=Wrap  en=off  latency=0  use_behavioral_HDL=off  opt=Speed  use_embedded=on  optimum_pipeline=off  pipeline=on  use_rpm=on  placement_style=Triangular  XmcBlockStatus=1  maskContainerNames=group1  block_type=mult  block_config=sysgen:Mult_config  block_width=598  block_height=876
  Out1 : Outport
  wires:
  Delay3/1 -> Mult4/2, Delay4/1
  Mult2/1 -> AddSub2/1
  In1/1 -> Mult/2, Delay/1
  Constant6/1 -> Mult6/1
  Delay5/1 -> Mult6/2, Delay6/1
  Constant7/1 -> Mult7/1
  Delay1/1 -> Mult2/2, Delay2/1
  Delay/1 -> Mult1/2, Delay1/1
  AddSub7/1 -> Out1/1
  Delay2/1 -> Mult3/2, Delay3/1
  AddSub4/1 -> AddSub5/2
  Delay6/1 -> Mult7/2
  Mult3/1 -> AddSub3/1
  Constant5/1 -> Mult5/1
  AddSub1/1 -> AddSub2/2
  Delay4/1 -> Mult5/2, Delay5/1
  Constant2/1 -> Mult2/1
  Mult7/1 -> AddSub7/1
  Mult1/1 -> AddSub1/1
  Mult6/1 -> AddSub6/1
  AddSub5/1 -> AddSub6/2
  Mult4/1 -> AddSub4/1
  AddSub3/1 -> AddSub4/2
  Constant3/1 -> Mult3/1
  Constant/1 -> Mult/1
  Mult5/1 -> AddSub5/1
  AddSub2/1 -> AddSub3/2
  Constant4/1 -> Mult4/1
  Mult/1 -> AddSub1/2
  AddSub6/1 -> AddSub7/2
  Constant1/1 -> Mult1/1

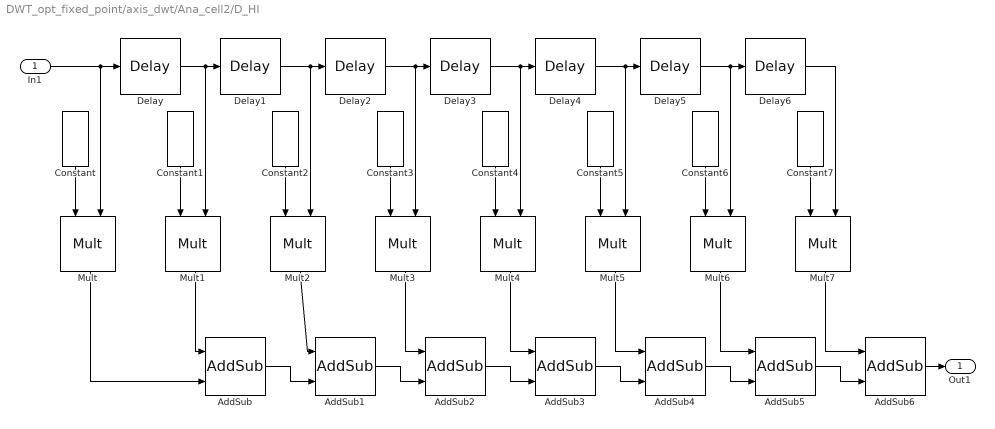
== system DWT_opt_fixed_point/axis_dwt/Ana_cell2/D_HI ==
  In1 : Inport
  AddSub{,1..6} (7 alike) : hdlBasic/AddSub  mode=Addition  use_carryin=off  use_carryout=off  en=off  latency=0  precision=User Defined  arith_type="Signed  (2's comp)"  n_bits=18  bin_pt=16  quantization=Truncate  overflow=Wrap  use_behavioral_HDL=off  hw_selection=Fabric  pipelined=off  XmcBlockStatus=1  maskContainerNames=tabcontainer1  block_type=addsub  block_config=sysgen:Addsub_config
  Constant : hdlBasic/Constant  const=-0.23037781330885523  gui_display_data_type=Fixed-point  arith_type=Signed (2's comp)  n_bits=16  bin_pt=14  preci_type=Single  exp_width=8  frac_width=24  explicit_period=off  period=1  XmcBlockStatus=1  maskContainerNames=tabcontainer1  block_type=constant  block_config=sysgen:Constant_config
  Constant1 : hdlBasic/Constant  const=0.7148465705525415  gui_display_data_type=Fixed-point  arith_type=Signed (2's comp)  n_bits=16  bin_pt=14  preci_type=Single  exp_width=8  frac_width=24  explicit_period=off  period=1  XmcBlockStatus=1  maskContainerNames=tabcontainer1  block_type=constant  block_config=sysgen:Constant_config
  Constant2 : hdlBasic/Constant  const=-0.6308807679295904  gui_display_data_type=Fixed-point  arith_type=Signed (2's comp)  n_bits=16  bin_pt=14  preci_type=Single  exp_width=8  frac_width=24  explicit_period=off  period=1  XmcBlockStatus=1  maskContainerNames=tabcontainer1  block_type=constant  block_config=sysgen:Constant_config
  Constant3 : hdlBasic/Constant  const=-0.02798376941698385  gui_display_data_type=Fixed-point  arith_type=Signed (2's comp)  n_bits=16  bin_pt=14  preci_type=Single  exp_width=8  frac_width=24  explicit_period=off  period=1  XmcBlockStatus=1  maskContainerNames=tabcontainer1  block_type=constant  block_config=sysgen:Constant_config
  Constant4 : hdlBasic/Constant  const=0.18703481171888114  gui_display_data_type=Fixed-point  arith_type=Signed (2's comp)  n_bits=16  bin_pt=14  preci_type=Single  exp_width=8  frac_width=24  explicit_period=off  period=1  XmcBlockStatus=1  maskContainerNames=tabcontainer1  block_type=constant  block_config=sysgen:Constant_config
  Constant5 : hdlBasic/Constant  const=0.030841381835986965  gui_display_data_type=Fixed-point  arith_type=Signed (2's comp)  n_bits=16  bin_pt=14  preci_type=Single  exp_width=8  frac_width=24  explicit_period=off  period=1  XmcBlockStatus=1  maskContainerNames=tabcontainer1  block_type=constant  block_config=sysgen:Constant_config
  Constant6 : hdlBasic/Constant  const=-0.032883011666982945  gui_display_data_type=Fixed-point  arith_type=Signed (2's comp)  n_bits=16  bin_pt=14  preci_type=Single  exp_width=8  frac_width=24  explicit_period=off  period=1  XmcBlockStatus=1  maskContainerNames=tabcontainer1  block_type=constant  block_config=sysgen:Constant_config
  Constant7 : hdlBasic/Constant  const=-0.010597401784997278  gui_display_data_type=Fixed-point  arith_type=Signed (2's comp)  n_bits=16  bin_pt=14  preci_type=Single  exp_width=8  frac_width=24  explicit_period=off  period=1  XmcBlockStatus=1  maskContainerNames=tabcontainer1  block_type=constant  block_config=sysgen:Constant_config
  Delay{,1..6} (7 alike) : hdlBasic/Delay  rst=off  en=off  latency=1  reg_retiming=off  XmcBlockStatus=1  maskContainerNames=group1  block_type=delay  block_config=sysgen:Delay_config
  Mult{,1..7} (8 alike) : hdlBasic/Mult  precision=User Defined  arith_type="Signed  (2's comp)"  n_bits=18  bin_pt=16  quantization=Truncate  overflow=Wrap  en=off  latency=0  use_behavioral_HDL=off  opt=Speed  use_embedded=on  optimum_pipeline=off  pipeline=on  use_rpm=on  placement_style=Triangular  XmcBlockStatus=1  maskContainerNames=group1  block_type=mult  block_config=sysgen:Mult_config  block_width=598  block_height=876
  Out1 : Outport
  wires:
  Delay3/1 -> Mult4/2, Delay4/1
  Mult2/1 -> AddSub1/1
  In1/1 -> Mult/2, Delay/1
  Constant6/1 -> Mult6/1
  Delay5/1 -> Mult6/2, Delay6/1
  Constant7/1 -> Mult7/1
  Delay1/1 -> Mult2/2, Delay2/1
  Delay/1 -> Mult1/2, Delay1/1
  AddSub6/1 -> Out1/1
  Delay2/1 -> Mult3/2, Delay3/1
  AddSub3/1 -> AddSub4/2
  Delay6/1 -> Mult7/2
  Mult3/1 -> AddSub2/1
  Constant5/1 -> Mult5/1
  AddSub/1 -> AddSub1/2
  Delay4/1 -> Mult5/2, Delay5/1
  Constant2/1 -> Mult2/1
  Mult7/1 -> AddSub6/1
  Mult1/1 -> AddSub/1
  Mult6/1 -> AddSub5/1
  AddSub4/1 -> AddSub5/2
  Mult4/1 -> AddSub3/1
  AddSub2/1 -> AddSub3/2
  Constant3/1 -> Mult3/1
  Constant/1 -> Mult/1
  Mult5/1 -> AddSub4/1
  AddSub1/1 -> AddSub2/2
  Constant4/1 -> Mult4/1
  Mult/1 -> AddSub/2
  AddSub5/1 -> AddSub6/2
  Constant1/1 -> Mult1/1
